simulink model "teleop"  (R2015a)
settings: Solver=ode45  StartTime=0.0  StopTime=20  RelTol=1e-3
values from neighbouring files (symbols this model uses):
  A_master = [0 1; 0 -Bm/Mm]    [teleop_test.m]
  A_slave = [0 1; 0 -Bs/Ms]    [teleop_test.m]
  B_master = [0; 1/Mm]    [teleop_test.m]
  B_slave = [0; 1/Ms]    [teleop_test.m]
  C_master = [1 0; 0 1]    [teleop_test.m]
  C_slave = [1 0; 0 1]    [teleop_test.m]
  D_master = [0; 0]    [teleop_test.m]
  D_slave = [0; 0]    [teleop_test.m]
  De = 0    [teleop_test.m]
  K = output.P    [master_test.m]    (also in teleop_test.m = output.h2)
  Ke = 0    [teleop_test.m]
  Me = 0    [teleop_test.m]
  Xe = 9    [teleop_test.m]
libraries: simulink x1
settings Model: Creator=enrico-giordano  LastModifiedBy=enrico-giordano

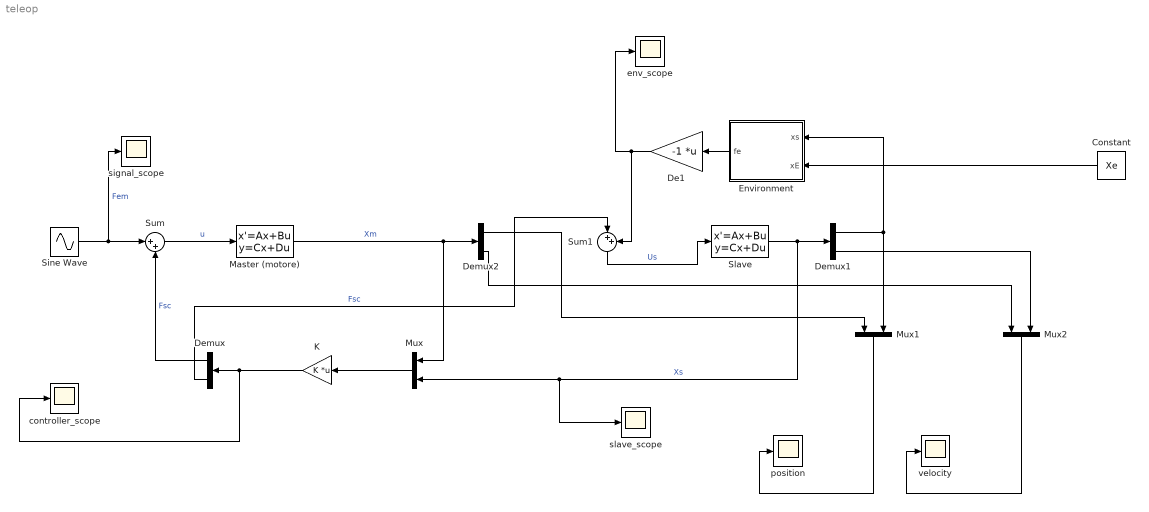
== system teleop ==
  Constant : Constant  Value=Xe
  De1 : Gain  Gain=-1  Multiplication=Matrix(K*u)
  Demux : Demux  Outputs=2
  Demux1 : Demux  Outputs=2
  Demux2 : Demux  Outputs=2
  Environment : Subsystem
  K : Gain  Gain=K  Multiplication=Matrix(K*u)
  Master (motore) : StateSpace  A=A_master  B=B_master  C=C_master  D=D_master  X0=0
  Mux : Mux  Inputs=2
  Mux1 : Mux  Inputs=2
  Mux2 : Mux  Inputs=2
  Sine Wave : Sin  Amplitude=10  SampleTime=0
  Slave : StateSpace  A=A_slave  B=B_slave  C=C_slave  D=D_slave  X0=0
  Sum : Sum  Inputs=|++
  Sum1 : Sum  Inputs=|++
  controller_scope : Scope
      settings: TimeRange=10  YMin=-0.6000000000000001  YMax=0.2  SaveName=ScopeData3
  env_scope : Scope
      settings: TimeRange=10  YMin=-1  YMax=2  SaveName=ScopeData4
  position : Scope
      settings: TimeRange=10  YMin=6.9  YMax=9.1  SaveName=ScopeData6
  signal_scope : Scope
      settings: TimeRange=10  YMin=-10  YMax=10
  slave_scope : Scope
      settings: TimeRange=10  YMin=-0.6000000000000001  YMax=0.2
  velocity : Scope
      settings: TimeRange=10  YMin=-1  YMax=2  SaveName=ScopeData7
  wires:
  Sum/1 -> Master (motore)/1  "u"
  Sine Wave/1 -> signal_scope/1, Sum/1  "Fem"
  Mux/1 -> K/1
  Master (motore)/1 -> Demux2/1, Mux/1  "Xm"
  Demux/2 -> Sum1/1  "Fsc"
  Sum1/1 -> Slave/1  "Us"
  Slave/1 -> slave_scope/1, Mux/2, Demux1/1  "Xs"
  De1/1 -> env_scope/1, Sum1/2
  Constant/1 -> Environment/2(xE)
  Environment/1(fe) -> De1/1
  Demux1/1 -> Mux1/2, Environment/1(xs)
  Demux/1 -> Sum/2  "Fsc"
  Demux2/1 -> Mux1/1
  Mux1/1 -> position/1
  Demux2/2 -> Mux2/1
  Demux1/2 -> Mux2/2
  Mux2/1 -> velocity/1
  K/1 -> controller_scope/1, Demux/1

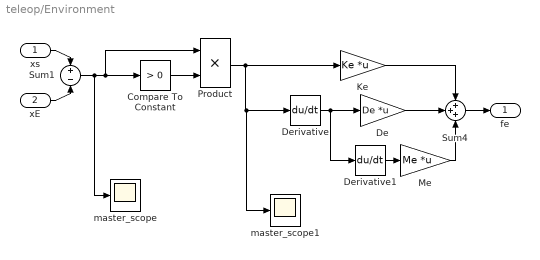
== system teleop/Environment ==
  xs : Inport
  xE : Inport  Port=2
  Compare To Constant : simulink/Logic and Bit Operations/Compare To Constant  relop=>  const=0  OutDataTypeStr=uint8  ZeroCross=off
  De : Gain  Gain=De  Multiplication=Matrix(K*u)
  Derivative : Derivative
  Derivative1 : Derivative
  Ke : Gain  Gain=Ke  Multiplication=Matrix(K*u)
  Me : Gain  Gain=Me  Multiplication=Matrix(K*u)
  Product : Product  RndMeth=Zero
  Sum1 : Sum  Inputs=+|-
  Sum4 : Sum  Inputs=+++
  master_scope : Scope
      settings: TimeRange=10  YMin=-1  YMax=2  SaveName=ScopeData5
  master_scope1 : Scope
      settings: TimeRange=10  YMin=-1  YMax=2  SaveName=ScopeData8
  fe : Outport
  wires:
  Compare To Constant/1 -> Product/2
  Sum1/1 -> master_scope/1, Compare To Constant/1, Product/1
  Product/1 -> Ke/1, master_scope1/1, Derivative/1
  Derivative/1 -> De/1, Derivative1/1
  Derivative1/1 -> Me/1
  Ke/1 -> Sum4/1
  De/1 -> Sum4/2
  Me/1 -> Sum4/3
  xs/1 -> Sum1/1
  xE/1 -> Sum1/2
  Sum4/1 -> fe/1
